simulink model "pHSystemRead"  (R2016b)
settings: Solver=FixedStepDiscrete  StartTime=0.0  StopTime=500  FixedStep=1  RelTol=1e-3  EnableMultiTasking=on
libraries: EEE481Arduino x2
settings Model: ExtModeTrigDuration=2  Creator=rsjoshi1  LastModifiedBy=rsjoshi1
settings OptimizationCC: LifeSpan=1  MaxStackSize=64
settings DebuggingCC: SFUnexpectedBacktrackingDiag=warning  SFNoUnconditionalDefaultTransitionDiag=warning  SFExecutionAtInitializationDiag=none
settings HardwareCC: ProdBitPerPointer=32  ProdBitPerSizeT=32  ProdBitPerPtrDiffT=32  ProdLargestAtomicInteger=Long  ProdLargestAtomicFloat=Double  ProdWordSize=32  ProdHWDeviceType=ARM Compatible->ARM Cortex
settings RTWCC: SystemTargetFile=ert.tlc  HardwareBoard=Arduino Due  TLCOptions=-aInlineSetEventsForThisBaseRateFcn=TLC_FALSE -aSuppressMultiTaskScheduler=TLC_FALSE -aRateBasedStepFcn=1  TemplateMakefile=ert_default_tmf  Description=Embedded Coder  GenerateReport=on  Toolchain=Arduino ARM v1.6.7  BuildConfiguration=Faster Runs  IncludeHyperlinkInReport=on  LaunchReport=on  GenerateTraceInfo=on  GenerateTraceReport=on  GenerateTraceReportSl=on  GenerateTraceReportSf=on  GenerateTraceReportEml=on
settings CodeAppCC: ForceParamTrailComments=on  IgnoreCustomStorageClasses=off  OperatorAnnotations=on  SimulinkDataObjDesc=on  SFDataObjDesc=on  MATLABFcnDesc=on  InsertBlockDesc=on  MATLABSourceComments=on
settings ERTTargetCC: SupportContinuousTime=on  SupportVariableSizeSignals=on
settings ConfigComp: CovMetricSettings=dw  CovHtmlReporting=on  CovSaveCumulativeToWorkspaceVar=on  CovSaveSingleToWorkspaceVar=on  CovExternalEMLEnable=off

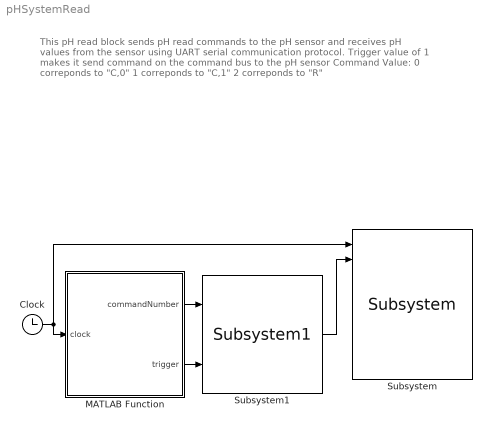
== system pHSystemRead ==
  note: This pH read block sends pH read commands to the pH sensor and receives pH values from the sensor using UART serial communication protocol. Trigger value of 1 makes it send command on the command bus to the pH sensor
      |
      | Command Value: 0 correponds to "C,0"
      | 1 correponds to "C,1"
      | 2 correponds to "R"
  Clock : Clock
  MATLAB Function : MATLAB Function  TreatAsAtomicUnit=on
  Subsystem : EEE481Arduino/Subsystem  Tsa=1  rate=0  per=0
  Subsystem1 : EEE481Arduino/Subsystem1  PortNum=2  Tsa=0
  wires:
  MATLAB Function/1(commandNumber) -> Subsystem1/1
  Clock/1 -> Subsystem/1, MATLAB Function/1(clock)
  MATLAB Function/2(trigger) -> Subsystem1/2
  Subsystem1/1 -> Subsystem/2

== matlab function pHSystemRead/MATLAB Function ==
  data: clock input; commandNumber output; trigger output
function [commandNumber,trigger] = QueryPHSensor(clock)
%#codegen
if(clock<2)
    commandNumber=int8(1);
elseif(clock>=100&&clock<200)
    commandNumber=int8(0);
else
    commandNumber=int8(2);
end
if(clock<2||clock==100||clock>=200)
    trigger=int8(1);
else
    trigger=int8(0);
end
end
